simulink model "a5_real_control_pid"  (R2023b)
settings: Solver=FixedStepAuto  StartTime=0.0  StopTime=inf  FixedStep=0.01  RelTol=1e-3  EnableMultiTasking=on
undefined symbols (not defined in the file): dev, Main, pid_y_i, pwm_output0
libraries: slpidlib x11, simulink x6, px4Sensorslib x5, px4lib x1, px4uORBlib x1
(part 2 of 2)

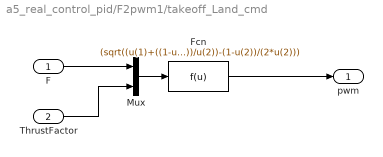
== system a5_real_control_pid/F2pwm1/takeoff_Land_cmd ==
  F : Inport
  ThrustFactor : Inport  Port=2
  Fcn : Fcn  Expr=(sqrt((u(1)+((1-u(2))^2)/(4*u(2)))/u(2))-(1-u(2))/(2*u(2)))
  Mux : Mux  Inputs=2
  pwm : Outport  OutDataTypeStr=boolean  VectorParamsAs1DForOutWhenUnconnected=off
  wires:
  Fcn/1 -> pwm/1
  Mux/1 -> Fcn/1
  F/1 -> Mux/1
  ThrustFactor/1 -> Mux/2

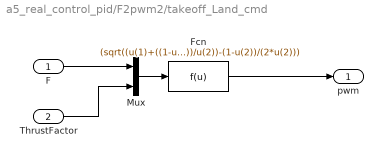
== system a5_real_control_pid/F2pwm2/takeoff_Land_cmd ==
  F : Inport
  ThrustFactor : Inport  Port=2
  Fcn : Fcn  Expr=(sqrt((u(1)+((1-u(2))^2)/(4*u(2)))/u(2))-(1-u(2))/(2*u(2)))
  Mux : Mux  Inputs=2
  pwm : Outport  OutDataTypeStr=boolean  VectorParamsAs1DForOutWhenUnconnected=off
  wires:
  Fcn/1 -> pwm/1
  Mux/1 -> Fcn/1
  F/1 -> Mux/1
  ThrustFactor/1 -> Mux/2

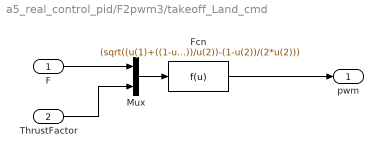
== system a5_real_control_pid/F2pwm3/takeoff_Land_cmd ==
  F : Inport
  ThrustFactor : Inport  Port=2
  Fcn : Fcn  Expr=(sqrt((u(1)+((1-u(2))^2)/(4*u(2)))/u(2))-(1-u(2))/(2*u(2)))
  Mux : Mux  Inputs=2
  pwm : Outport  OutDataTypeStr=boolean  VectorParamsAs1DForOutWhenUnconnected=off
  wires:
  Fcn/1 -> pwm/1
  Mux/1 -> Fcn/1
  F/1 -> Mux/1
  ThrustFactor/1 -> Mux/2

== system a5_real_control_pid/RC_cmd/ArmingControl ==
  ch7 : Inport
  Compare To Constant1 : simulink/Logic and Bit Operations/Compare To Constant  relop=>=  const=uint16(1800)  OutDataTypeStr=boolean
  ARM Control : Outport  OutDataTypeStr=boolean  VectorParamsAs1DForOutWhenUnconnected=off
  wires:
  Compare To Constant1/1 -> ARM Control/1
  ch7/1 -> Compare To Constant1/1

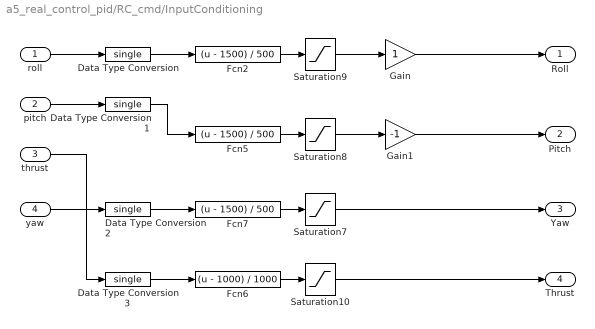
== system a5_real_control_pid/RC_cmd/InputConditioning ==
  roll : Inport
  pitch : Inport  Port=2
  thrust : Inport  Port=3
  yaw : Inport  Port=4
  Data Type Conversion{,1..3} (4 alike) : DataTypeConversion  OutDataTypeStr=single  SaturateOnIntegerOverflow=off  RndMeth=Floor
  Fcn2 : Fcn  Expr=(u - 1500) / 500
  Fcn5 : Fcn  Expr=(u - 1500) / 500
  Fcn6 : Fcn  Expr=(u - 1000) / 1000
  Fcn7 : Fcn  Expr=(u - 1500) / 500
  Gain : Gain
  Gain1 : Gain  Gain=-1
  Saturation10 : Saturate  UpperLimit=1  LowerLimit=0
  Saturation7 : Saturate  UpperLimit=1  LowerLimit=-1
  Saturation8 : Saturate  UpperLimit=1  LowerLimit=-1
  Saturation9 : Saturate  UpperLimit=1  LowerLimit=-1
  Roll : Outport  VectorParamsAs1DForOutWhenUnconnected=off
  Pitch : Outport  Port=2  VectorParamsAs1DForOutWhenUnconnected=off
  Yaw : Outport  Port=3  VectorParamsAs1DForOutWhenUnconnected=off
  Thrust : Outport  Port=4  VectorParamsAs1DForOutWhenUnconnected=off
  wires:
  Data Type Conversion3/1 -> Fcn6/1
  Data Type Conversion2/1 -> Fcn7/1
  Data Type Conversion1/1 -> Fcn5/1
  Data Type Conversion/1 -> Fcn2/1
  roll/1 -> Data Type Conversion/1
  pitch/1 -> Data Type Conversion1/1
  yaw/1 -> Data Type Conversion2/1
  Fcn7/1 -> Saturation7/1
  Saturation9/1 -> Gain/1
  Fcn5/1 -> Saturation8/1
  Fcn2/1 -> Saturation9/1
  thrust/1 -> Data Type Conversion3/1
  Fcn6/1 -> Saturation10/1
  Saturation8/1 -> Gain1/1
  Saturation7/1 -> Yaw/1
  Saturation10/1 -> Thrust/1
  Gain/1 -> Roll/1
  Gain1/1 -> Pitch/1

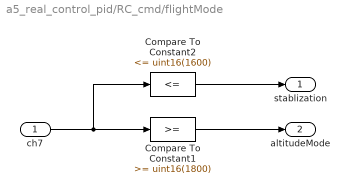
== system a5_real_control_pid/RC_cmd/flightMode ==
  ch7 : Inport
  Compare To Constant1 : simulink/Logic and Bit Operations/Compare To Constant  relop=>=  const=uint16(1800)  OutDataTypeStr=boolean
  Compare To Constant2 : simulink/Logic and Bit Operations/Compare To Constant  relop=<=  const=uint16(1600)  OutDataTypeStr=boolean
  stablization : Outport  OutDataTypeStr=boolean  VectorParamsAs1DForOutWhenUnconnected=off
  altitudeMode : Outport  Port=2  OutDataTypeStr=boolean  VectorParamsAs1DForOutWhenUnconnected=off
  wires:
  ch7/1 -> Compare To Constant2/1, Compare To Constant1/1
  Compare To Constant1/1 -> altitudeMode/1
  Compare To Constant2/1 -> stablization/1

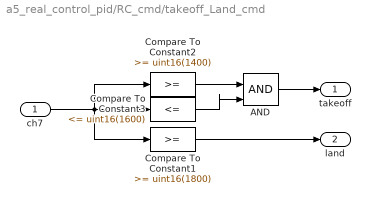
== system a5_real_control_pid/RC_cmd/takeoff_Land_cmd ==
  ch7 : Inport
  AND : Logic  IconShape=distinctive  AllPortsSameDT=off  OutDataTypeStr=boolean
  Compare To Constant1 : simulink/Logic and Bit Operations/Compare To Constant  relop=>=  const=uint16(1800)  OutDataTypeStr=boolean
  Compare To Constant2 : simulink/Logic and Bit Operations/Compare To Constant  relop=>=  const=uint16(1400)  OutDataTypeStr=boolean
  Compare To Constant3 : simulink/Logic and Bit Operations/Compare To Constant  relop=<=  const=uint16(1600)  OutDataTypeStr=boolean
  takeoff : Outport  OutDataTypeStr=boolean  VectorParamsAs1DForOutWhenUnconnected=off
  land : Outport  Port=2  OutDataTypeStr=boolean  VectorParamsAs1DForOutWhenUnconnected=off
  wires:
  Compare To Constant1/1 -> land/1
  ch7/1 -> Compare To Constant1/1, Compare To Constant3/1, Compare To Constant2/1
  Compare To Constant2/1 -> AND/1
  Compare To Constant3/1 -> AND/2
  AND/1 -> takeoff/1

== matlab function a5_real_control_pid/Subsystem3/MATLAB Function1 ==
  data: phi input double; gain output double; theta input double
function gain = fcn(phi, theta)

gain = 1/(cos(phi) * cos(theta));

== matlab function a5_real_control_pid/fai_d&psi_dGenerator2 ==
  data: psi input double; phi_d output double; u1x input double; u1y input double; u1z input double; theta_d output double
function [phi_d, theta_d] = fcn(psi, u1x, u1y, u1z)

% fai_d = atan((y_d - y)/(x_d - x));
% theta_d = atan((z_d - z)/(((x_d - x)^2 + (y_d - y)^2)^(1/2)));
phi_d = -1 * atan((u1x * sin(psi) - u1y * cos(psi)) / u1z );
theta_d = -1 * atan((u1x * cos(psi) + u1y * sin(psi)) * cos(phi_d) / u1z );

== matlab function a5_real_control_pid/fai_d&psi_dGenerator3 ==
  data: u1 input double; F1 output double; u2 input double; u3 input double; u4 input double; F2 output double; F3 output; F4 output
function [F1,F2,F3,F4] = fcn(u1, u2, u3, u4)

L = 0.25; Km = 1;
convertMatrix = [1              1           1           1;
                 -L/sqrt(2)     L/sqrt(2)   L/sqrt(2)   -L/sqrt(2);
                 L/sqrt(2)      -L/sqrt(2)  L/sqrt(2)   -L/sqrt(2);
                 Km/sqrt(2)     Km/sqrt(2)  -Km/sqrt(2) -Km/sqrt(2)];
% convertMatrix_inv=[0.2500   -1.4142    1.4142    0.3536;
%                    0.2500    1.4142   -1.4142    0.3536;
%                    0.2500    1.4142    1.4142   -0.3536;
%                    0.2500   -1.4142   -1.4142   -0.3536]
%F = inv(convertMatrix) * [u1; u2; u3; u4];
F = convertMatrix \ [u1; u2; u3; u4];
F1 = F(1);
F2 = F(2);
F3 = F(3);
F4 = F(4);

% convertMatrix_ref = [-0.3536    0.3536    0.3536   -0.3536;
%                       0.3536   -0.3536    0.3536   -0.3536;
%                       0.2500    0.2500   -0.2500   -0.2500;
%                       0.2500    0.2500    0.2500    0.2500];
% convertMatrix_ref_inv = [-1/sqrt(2)       1/sqrt(2)   1 1;
%                           1/sqrt(2)      -1/sqrt(2)   1 1;
%                           1/sqrt(2)       1/sqrt(2)  -1 1;
%                          -1/sqrt(2)      -1/sqrt(2)  -1 1]

== matlab function a5_real_control_pid/quat2eul ==
  data: q input; phi output; theta output; psi output
function [phi,theta,psi] = quat2eul(q)

% Quaternion conversion to Euler angles based on the PX4 Firmware v1.10.2
% release.

phi = atan2(2*(q(1)*q(2) + q(3)* q(4)), q(1)^2 - q(2)^2 - q(3)^2 + q(4)^2);
theta = asin(-2*(q(2)*q(4) - q(1)*q(3)));
psi = atan2(2*(q(2)*q(3) + q(1)* q(4)), q(1)^2 + q(2)^2 - q(3)^2 - q(4)^2);

end
